simulink model "multi_model"  (R2016b)
settings: Solver=ode15s  StartTime=0.0  StopTime=inf  FixedStep=0.001  MaxStep=0.004  RelTol=1e-3
InitFcn:
  | kR_old=0;
  | kOm_old=0;
undefined symbols (not defined in the file): deg, rad, s
libraries: simulink x23, aerolibconvert2 x3, aerolibobsolete x1, aerolibtransform2 x1, aerolibatmos2 x1, aerolibnav x1, aerolibanimutils x1
(part 1 of 2)
settings Model: Creator=ADAM  LastModifiedBy=luminghua
settings SolverCC: ExtrapolationOrder=1
settings DataIOCC: MaxDataPoints=1  SaveFormat=Structure  SignalLoggingSaveFormat=ModelDataLogs  SaveOutput=off  SignalLogging=off  DSMLogging=off  SaveTime=off  OutputSaveName=model_out  SignalLoggingName=model_out
settings OptimizationCC: ExpressionDepthLimit=2147483647  LifeSpan=inf  SimCompilerOptimization=on
settings DebuggingCC: UnderspecifiedInitializationDetection=Classic  MergeDetectMultiDrivingBlocksExec=none  SolverPrmCheckMsg=warning  InheritedTsInSrcMsg=none  MultiTaskDSMMsg=warning  MultiTaskCondExecSysMsg=none  FcnCallInpInsideContextMsg=warning  UnconnectedInputMsg=none  UnconnectedOutputMsg=none  UnconnectedLineMsg=none  AllowSymbolicDim=off  StateNameClashWarn=warning  SFUnexpectedBacktrackingDiag=warning  SFNoUnconditionalDefaultTransitionDiag=warning  SFExecutionAtInitializationDiag=none
settings HardwareCC: ProdBitPerPointer=32  ProdBitPerSizeT=32  ProdBitPerPtrDiffT=32  ProdLargestAtomicFloat=None  ProdWordSize=32  ProdHWDeviceType=Generic->32-bit x86 compatible
settings ModelReferenceCC: PropagateSignalLabelsOutOfModel=off
settings CodeAppCC: MaxIdLength=95
settings GRTTargetCC: TargetLangStandard=C89/C90 (ANSI)  GeneratePreprocessorConditionals=Disable all
settings ConfigComp: CovMetricSettings=dw  CovHtmlReporting=on  CovSaveCumulativeToWorkspaceVar=on  CovSaveSingleToWorkspaceVar=on  CovExternalEMLEnable=off

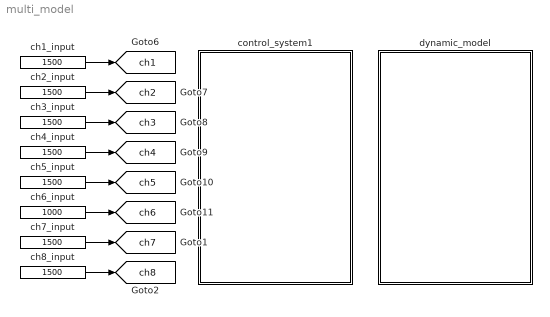
== system multi_model ==
  ch1_input : Constant  Value=1500  SampleTime=0.004
  ch2_input : Constant  Value=1500  SampleTime=0.004
  ch3_input : Constant  Value=1500  SampleTime=0.004
  ch4_input : Constant  Value=1500  SampleTime=0.004
  ch5_input : Constant  Value=1500  SampleTime=0.004
  ch6_input : Constant  Value=1000  SampleTime=0.004
  ch7_input : Constant  Value=1500  SampleTime=0.004
  ch8_input : Constant  Value=1500  SampleTime=0.004
  control_system1 : Subsystem
      mask Display: fprintf('Embedded Software')
  dynamic_model : Subsystem
      mask Display: fprintf('Dynamic Model');
  tag scope: ch1=global, ch2=global, ch3=global, ch4=global, ch5=global, ch6=global, ch7=global, ch8=global
  wires:
  ch3_input/1 -> [ch3]
  ch2_input/1 -> [ch2]
  ch1_input/1 -> [ch1]
  ch4_input/1 -> [ch4]
  ch5_input/1 -> [ch5]
  ch6_input/1 -> [ch6]
  ch7_input/1 -> [ch7]
  ch8_input/1 -> [ch8]

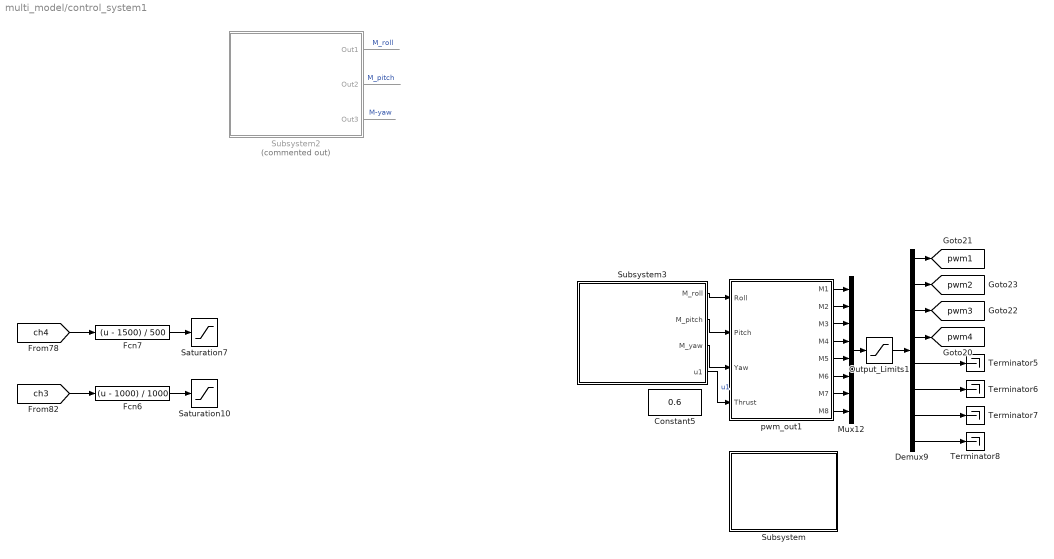
== system multi_model/control_system1 ==
  Constant5 : Constant  Value=0.6  SampleTime=0.004
  Demux9 : Demux  Outputs=8
  Fcn6 : Fcn  Expr=(u - 1000) / 1000
  Fcn7 : Fcn  Expr=(u - 1500) / 500
  Mux12 : Mux  Inputs=8
  Output_Limits1 : Saturate  UpperLimit=2000  LowerLimit=1000
  Saturation10 : Saturate  UpperLimit=1  LowerLimit=0
  Saturation7 : Saturate  UpperLimit=1  LowerLimit=-1
  Subsystem : Subsystem
      mask Display: disp('Test')
  Subsystem2 : Subsystem  Commented=on
      mask Display: disp( 'Attitude_controller  PID')
  Subsystem3 : Subsystem
      mask Display: disp('Attitude_controller distur');
  Terminator{5..8} (4 alike) : Terminator
  pwm_out1 : MATLAB Function  TreatAsAtomicUnit=on  SystemSampleTime=0.004
  tag scope: pwm1=global, pwm2=global, pwm3=global, pwm4=global
  wires:
  pwm_out1/8(M8) -> Mux12/8
  pwm_out1/7(M7) -> Mux12/7
  pwm_out1/6(M6) -> Mux12/6
  pwm_out1/5(M5) -> Mux12/5
  pwm_out1/4(M4) -> Mux12/4
  pwm_out1/3(M3) -> Mux12/3
  pwm_out1/2(M2) -> Mux12/2
  pwm_out1/1(M1) -> Mux12/1
  Mux12/1 -> Output_Limits1/1
  [ch4] -> Fcn7/1
  Fcn7/1 -> Saturation7/1
  Demux9/5 -> Terminator5/1
  Demux9/6 -> Terminator6/1
  Demux9/7 -> Terminator7/1
  Demux9/8 -> Terminator8/1
  Demux9/1 -> [pwm1]
  Demux9/2 -> [pwm2]
  Demux9/3 -> [pwm3]
  Demux9/4 -> [pwm4]
  [ch3] -> Fcn6/1
  Fcn6/1 -> Saturation10/1
  Output_Limits1/1 -> Demux9/1
  Subsystem3/4(u1) -> pwm_out1/4(Thrust)  "u1"
  Subsystem2/1(Out1) -> ?  "M_roll"
  Subsystem2/2(Out2) -> ?  "M_pitch"
  Subsystem2/3(Out3) -> ?  "M-yaw"
  Subsystem3/1(M_roll) -> pwm_out1/1(Roll)
  Subsystem3/2(M_pitch) -> pwm_out1/2(Pitch)
  Subsystem3/3(M_yaw) -> pwm_out1/3(Yaw)

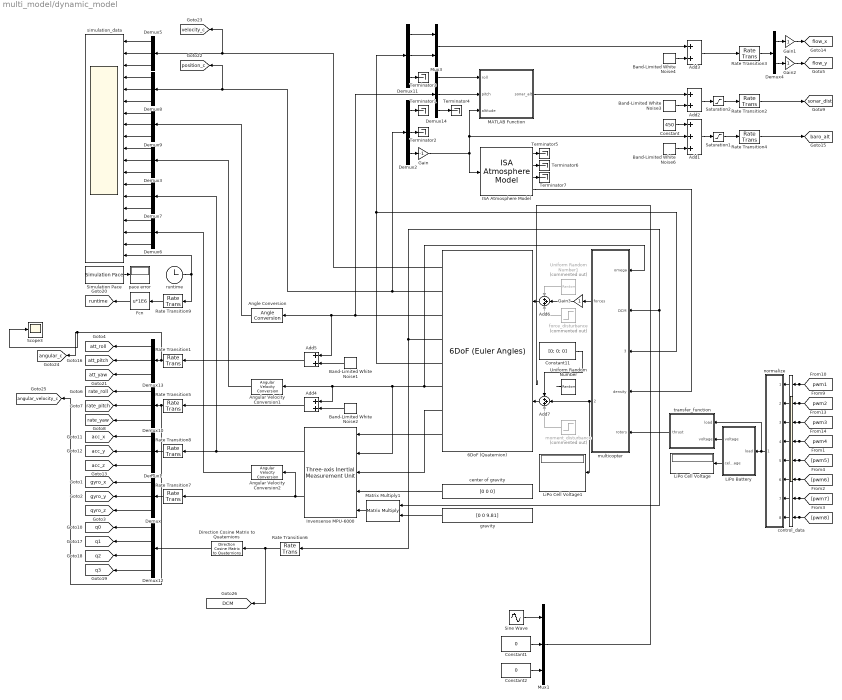
== system multi_model/dynamic_model ==
  6DoF (Quaternion) : aerolibobsolete/6DoF (Euler Angles)  units=Metric (MKS)  mtype=Fixed  rep=Quaternion  xme_0=[0 0 0]  Vm_0=[0 0 0]  eul_0=[0 0 0]  pm_0=[0 0 0]  mass_0=0.26  mass_e=0  mass_f=0  inertia=[0.00080, 0, 0; 0, 0.00065, 0; 0, 0, 0.0014]  inertia_e=eye(3)  inertia_f=eye(3)  k_quat=1.0
  Add1 : Sum  Inputs=+++
  Add{2..5} (4 alike) : Sum
  Add6 : Sum  Inputs=+++
  Add7 : Sum  Inputs=+++
  Angle Conversion : aerolibconvert2/Angle Conversion  IU=rad  OU=deg
  Angular Velocity Conversion1 : aerolibconvert2/Angular Velocity Conversion  IU=rad/s  OU=deg/s
  Angular Velocity Conversion2 : aerolibconvert2/Angular Velocity Conversion  IU=rad/s  OU=deg/s
  Band-Limited White Noise1 : simulink/Sources/Band-Limited White Noise  Cov=0.00000000015  Ts=0.004  seed=[243584]
  Band-Limited White Noise2 : simulink/Sources/Band-Limited White Noise  Cov=0.000000002  Ts=0.004  seed=[243584]
  Band-Limited White Noise3 : simulink/Sources/Band-Limited White Noise  Cov=0.000005  Ts=0.1  seed=[31841]
  Band-Limited White Noise4 : simulink/Sources/Band-Limited White Noise  Cov=0.000000003  Ts=0.0067  seed=[25481]
  Band-Limited White Noise6 : simulink/Sources/Band-Limited White Noise  Cov=0.0005  Ts=0.008  seed=[79648]
  Constant : Constant  Value=450
  Constant1 : Constant  Value=0  SampleTime=0.004
  Constant11 : Constant  Value=[0; 0; 0]  SampleTime=5
  Constant2 : Constant  Value=0  SampleTime=0.004
  Demux{,1..3,5..11,13..14} (13 alike) : Demux  Outputs=3
  Demux12 : Demux
  Demux4 : Demux  Outputs=2
  Direction Cosine Matrix to Quaternions : aerolibtransform2/Direction Cosine Matrix  to Quaternions
  Fcn : Fcn  Expr=u*1E6
      mask Display: fprintf('uS');
  Gain : Gain  Gain=-1
  Gain1 : Gain
  Gain2 : Gain
  Gain3 : Gain
  ISA Atmosphere Model : aerolibatmos2/ISA Atmosphere Model  custom=on  g=9.80665  gamma=1.4  R=287.0531  L=0.0065  h_trop=11000  h_strat=20000  rho0=1.225  P0=101325  T0=288.15  h0=0
  Invensense MPU-6000 : aerolibnav/Three-axis Inertial Measurement Unit  units=Metric (MKS)  imu=[0 0 0]  i_Ts=0.004  dtype_a=off  w_a=190  z_a=0.707  a_sf_cc=[0.98 0 0; 0 0.98 0; 0 0 0.98]  a_bias=[0 0 0]  a_sat="[-19.62  -19.62  -19.62 19.62 19.62 19.62]"  dtype_g=off  w_g=190  z_g=0.707  g_sf_cc=[.98 0 0; 0 .98 0; 0 0 .98]  g_bias=[0 0 0]  g_sens=[0 0 0]  g_sat="[-4.36  -4.36  -4.36 4.36 4.36 4.36]"  i_rand=on  i_seeds=[348631 366719 978432 189621 128794 214632]  i_pow=[0.0000005 0.0000005 0.0000005 0.000000002 0.000000002 0.000000002]
  LiPo Battery : MATLAB Function  TreatAsAtomicUnit=on  SystemSampleTime=0.004
  LiPo Cell Voltage : Display
  LiPo Cell Voltage1 : Display
  MATLAB Function : MATLAB Function  TreatAsAtomicUnit=on
  Matrix Multiply1 : Product  Multiplication=Matrix(*)
  Mux1 : Mux  Inputs=3
  Mux3 : Mux  Inputs=2
  Rate Transition{1,5..9} (6 alike) : RateTransition  OutPortSampleTime=0.004
  Rate Transition2 : RateTransition  OutPortSampleTime=0.1
  Rate Transition3 : RateTransition  OutPortSampleTime=0.0067
  Rate Transition4 : RateTransition  OutPortSampleTime=0.008
  Saturation1 : Saturate  UpperLimit=inf  LowerLimit=0
  Saturation2 : Saturate  UpperLimit=5  LowerLimit=0.3
  Scope3 : Scope
  Simulation Pace : aerolibanimutils/Simulation Pace  SimulationPace=1  SleepMode=MATLAB Thread  OutputPaceError=on  SampleTime=0.004
      settings: AttributesFormatString=%<SimulationPace> sec/sec
  Sine Wave : Sin  Amplitude=0.5  Frequency=0.01  SampleTime=0.004
  Terminator{1..7} (7 alike) : Terminator
  Uniform Random Number : UniformRandomNumber  Minimum=[-0.0005 -0.0005 -0.0001]  Maximum=[0.5 0.0005 0.0001]  SampleTime=5
  Uniform Random Number1 : UniformRandomNumber  Commented=on  Minimum=[-0.01 -0.01 -0.1]  Maximum=[0.01 0.01 0.1]  SampleTime=5
  center of gravity : Constant  Value=[0 0 0]
  control_data : Scope  NumInputPorts=8
  force_disturbance : Step  Commented=on  Time=5  Before=[0 0 0]  After=[0 0 0]
  gravity : Constant  Value=[0 0 9.81]
  moment_disturbance : Step  Commented=on  Time=5  Before=[0 0 0]  After=[0 0 0]
  multicopter : MATLAB Function  TreatAsAtomicUnit=on
  normalize : Subsystem
      mask Display:
      | port_label('input', 1, 'pwm1');
      | port_label('input', 2, 'pwm2');
      | port_label('input', 3, 'pwm3');
      | port_label('input', 4, 'pwm4');
      | port_label('input', 5, 'pwm5');
      | port_label('input', 6, 'pwm6');
      | port_label('input', 7, 'pwm7');
      | port_label('input', 8, 'pwm8');
  pace error : Display
  runtime : Clock
  simulation_data : Scope  NumInputPorts=19
  transfer_function : Subsystem
      mask Display: fprintf('Brushless Motors')
  tag scope: DCM=global, acc_x=global, acc_y=global, acc_z=global, angular_c=global, angular_velocity_c=global, att_pitch=global, att_roll=global, att_yaw=global, baro_alt=global, flow_x=global, flow_y=global, gyro_x=global, gyro_y=global, position_c=global, q0=global, q1=global, q2=global, q3=global, qyro_z=global, rate_pitch=global, rate_roll=global, rate_yaw=global, runtime=global, sonar_dist=global, velocity_c=global
  wires:
  6DoF (Quaternion)/7 -> Invensense MPU-6000/3
  Demux1/1 -> [acc_x]
  6DoF (Quaternion)/3 -> Demux14/1, Angle Conversion/1, Add5/1
  6DoF (Quaternion)/8 -> Invensense MPU-6000/1
  6DoF (Quaternion)/5 -> Demux11/1, multicopter/3(velocity)
  Demux9/1 -> simulation_data/7
  Demux9/2 -> simulation_data/8
  Demux3/1 -> simulation_data/10
  Demux3/2 -> simulation_data/11
  Demux3/3 -> simulation_data/12
  Demux7/1 -> simulation_data/13
  Demux7/2 -> simulation_data/14
  Demux7/3 -> simulation_data/15
  Demux/1 -> [gyro_x]
  Demux/2 -> [gyro_y]
  Demux/3 -> [qyro_z]
  Demux1/2 -> [acc_y]
  Demux5/1 -> simulation_data/1
  Demux5/2 -> simulation_data/2
  Demux5/3 -> simulation_data/3
  Demux8/1 -> simulation_data/4
  Demux8/2 -> simulation_data/5
  Demux8/3 -> simulation_data/6
  6DoF (Quaternion)/6 -> multicopter/1(omega), Invensense MPU-6000/2, Add4/1, Angular Velocity Conversion1/1
  Demux9/3 -> simulation_data/9
  Demux6/1 -> simulation_data/16
  Demux6/2 -> simulation_data/17
  Demux6/3 -> simulation_data/18
  Angular Velocity Conversion2/1 -> Demux6/1
  Demux1/3 -> [acc_z]
  Demux10/1 -> [rate_roll]
  Demux10/2 -> [rate_pitch]
  Demux10/3 -> [rate_yaw]
  Band-Limited White Noise2/1 -> Add4/2
  Add4/1 -> Rate Transition5/1
  Rate Transition5/1 -> [angular_velocity_c], Demux10/1
  6DoF (Quaternion)/4 -> Rate Transition6/1, Matrix Multiply1/1, multicopter/2(DCM)
  Simulation Pace/1 -> pace error/1
  6DoF (Quaternion)/1 -> Demux5/1, [velocity_c]
  6DoF (Quaternion)/2 -> Demux2/1, Demux8/1, [position_c]
  Angle Conversion/1 -> Demux9/1
  Angular Velocity Conversion1/1 -> Demux3/1
  Invensense MPU-6000/1 -> Rate Transition8/1, Demux7/1
  Invensense MPU-6000/2 -> Rate Transition7/1, Angular Velocity Conversion2/1
  runtime/1 -> simulation_data/19, Rate Transition9/1
  Rate Transition7/1 -> Demux/1
  Rate Transition8/1 -> Demux1/1
  Direction Cosine Matrix to Quaternions/1 -> Demux12/1
  [pwm1] -> normalize/1(pwm1), control_data/1
  [pwm2] -> normalize/2(pwm2), control_data/2
  [pwm3] -> normalize/3(pwm3), control_data/3
  [pwm4] -> normalize/4(pwm4), control_data/4
  [pwm5] -> normalize/5(pwm5), control_data/5
  [pwm6] -> normalize/6(pwm6), control_data/6
  [pwm7] -> normalize/7(pwm7), control_data/7
  [pwm8] -> normalize/8(pwm8), control_data/8
  Demux12/4 -> [q3]
  Demux12/3 -> [q2]
  Demux12/2 -> [q1]
  Demux12/1 -> [q0]
  Fcn/1 -> [runtime]
  Rate Transition9/1 -> Fcn/1
  normalize/1(normalized_signals) -> transfer_function/1(load), LiPo Battery/1(load)
  LiPo Battery/1(voltage) -> transfer_function/2(voltage)
  transfer_function/1(thrust) -> multicopter/5(rotors)
  LiPo Battery/2(cell_voltage) -> LiPo Cell Voltage/1
  Demux13/1 -> [att_roll]
  Demux13/2 -> [att_pitch]
  Demux13/3 -> [att_yaw]
  Rate Transition1/1 -> Scope3/1, [angular_c], Demux13/1
  Band-Limited White Noise1/1 -> Add5/2
  Add5/1 -> Rate Transition1/1
  Add6/1 -> 6DoF (Quaternion)/1
  Add7/1 -> 6DoF (Quaternion)/2
  center of gravity/1 -> Invensense MPU-6000/4
  gravity/1 -> Matrix Multiply1/2
  Matrix Multiply1/1 -> Invensense MPU-6000/5
  moment_disturbance/1 -> Add7/3
  force_disturbance/1 -> Add6/3
  multicopter/1(forces) -> Gain3/1
  Uniform Random Number1/1 -> Add6/1
  Uniform Random Number/1 -> ?
  Rate Transition3/1 -> Demux4/1
  Add3/1 -> Rate Transition3/1
  Demux2/3 -> Gain/1
  Gain/1 -> ISA Atmosphere Model/1, MATLAB Function/3(altitude), Add1/2
  Demux2/2 -> Terminator2/1
  Demux2/1 -> Terminator1/1
  Demux11/1 -> Mux3/1
  Demux11/2 -> Mux3/2
  Demux11/3 -> Terminator3/1
  Rate Transition2/1 -> [sonar_dist]
  Rate Transition4/1 -> [baro_alt]
  Saturation1/1 -> Rate Transition4/1
  Saturation2/1 -> Rate Transition2/1
  Add1/1 -> Saturation1/1
  MATLAB Function/1(sonar_alt) -> Add2/1
  Band-Limited White Noise3/1 -> Add2/2
  Add2/1 -> Saturation2/1
  Band-Limited White Noise4/1 -> Add3/2
  Band-Limited White Noise6/1 -> Add1/3
  Constant/1 -> Add1/1
  Mux3/1 -> Add3/1
  Demux4/2 -> Gain2/1
  Demux4/1 -> Gain1/1
  Gain1/1 -> [flow_x]
  Gain2/1 -> [flow_y]
  Demux14/2 -> MATLAB Function/2(pitch)
  Demux14/1 -> MATLAB Function/1(roll)
  Demux14/3 -> Terminator4/1
  ISA Atmosphere Model/3 -> Terminator7/1
  ISA Atmosphere Model/2 -> Terminator6/1
  ISA Atmosphere Model/1 -> Terminator5/1
  ISA Atmosphere Model/4 -> multicopter/4(density)
  Constant11/1 -> Add7/1
  multicopter/2(moments) -> Add7/2, LiPo Cell Voltage1/1
  Gain3/1 -> Add6/2
  Sine Wave/1 -> Mux1/1
  Constant1/1 -> Mux1/2
  Constant2/1 -> Mux1/3
  Mux1/1 -> ?
  Rate Transition6/1 -> [DCM], Direction Cosine Matrix to Quaternions/1

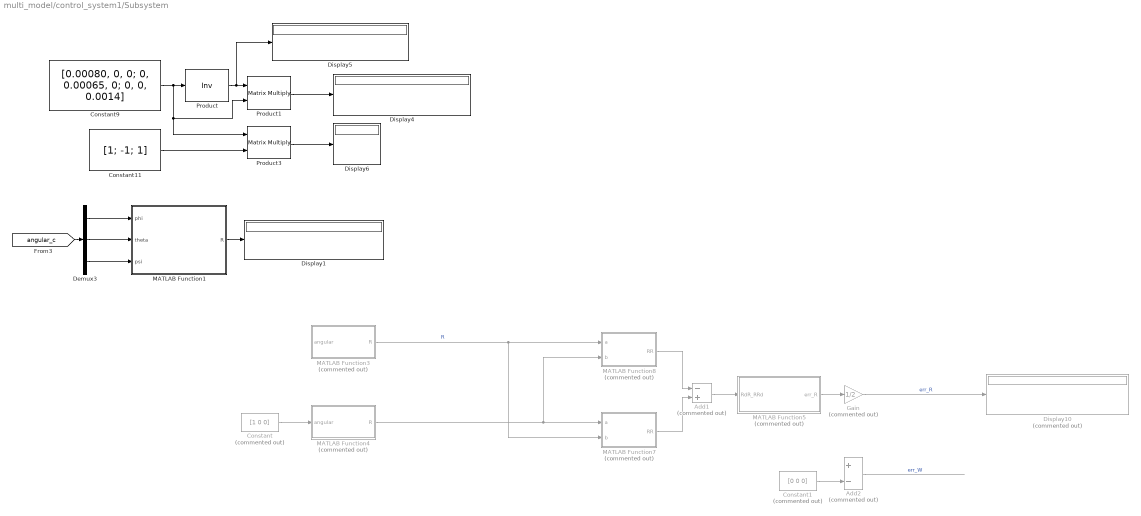
== system multi_model/control_system1/Subsystem ==
  Add1 : Sum  Commented=on  Inputs=-+
  Add2 : Sum  Commented=on  Inputs=+-
  Constant : Constant  Commented=on  Value=[1 0 0]
  Constant1 : Constant  Commented=on  Value=[0 0 0]
  Constant11 : Constant  Value=[1; -1; 1]  SampleTime=0.004
  Constant9 : Constant  Value=[0.00080, 0, 0; 0, 0.00065, 0; 0, 0, 0.0014]  SampleTime=0.004
  Demux3 : Demux  Outputs=3
  Display{1,4..6} (4 alike) : Display
  Display10 : Display  Commented=on
  Gain : Gain  Commented=on  Gain=1/2
  MATLAB Function1 : MATLAB Function  TreatAsAtomicUnit=on
  MATLAB Function3 : MATLAB Function  Commented=on  TreatAsAtomicUnit=on
  MATLAB Function4 : MATLAB Function  Commented=on  TreatAsAtomicUnit=on
  MATLAB Function5 : MATLAB Function  Commented=on  TreatAsAtomicUnit=on
  MATLAB Function7 : MATLAB Function  Commented=on  TreatAsAtomicUnit=on
  MATLAB Function8 : MATLAB Function  Commented=on  TreatAsAtomicUnit=on
  Product : Product  Inputs=/  Multiplication=Matrix(*)
  Product1 : Product  Multiplication=Matrix(*)
  Product3 : Product  Multiplication=Matrix(*)
  wires:
  ? -> Add2/1
  ? -> MATLAB Function3/1(angular)
  MATLAB Function7/1(RR) -> Add1/2
  Add1/1 -> MATLAB Function5/1(RdR_RRd)
  Constant/1 -> MATLAB Function4/1(angular)
  Gain/1 -> Display10/1  "err_R"
  MATLAB Function3/1(R) -> MATLAB Function8/1(a), MATLAB Function7/2(b)  "R"
  MATLAB Function5/1(err_R) -> Gain/1
  MATLAB Function8/1(RR) -> Add1/1
  MATLAB Function4/1(R) -> MATLAB Function8/2(b), MATLAB Function7/1(a)
  Constant1/1 -> Add2/2
  Product/1 -> Product1/1, Display5/1
  Constant11/1 -> Product3/2
  Constant9/1 -> Product3/1, Product1/2, Product/1
  Add2/1 -> ?  "err_W"
  Product3/1 -> Display6/1
  Product1/1 -> Display4/1
  MATLAB Function1/1(R) -> Display1/1
  Demux3/2 -> MATLAB Function1/2(theta)
  Demux3/1 -> MATLAB Function1/1(phi)
  Demux3/3 -> MATLAB Function1/3(psi)
  [angular_c] -> Demux3/1

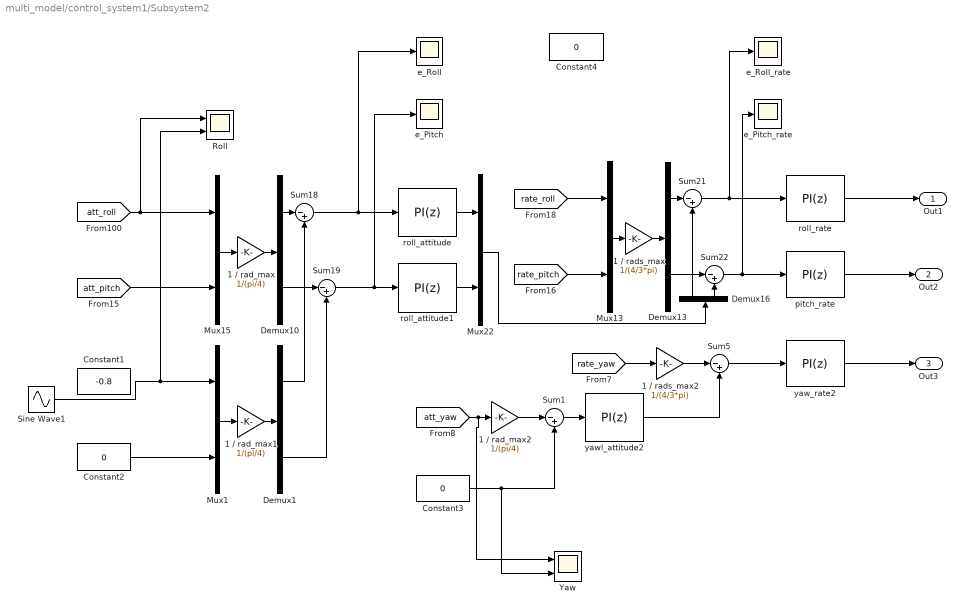
== system multi_model/control_system1/Subsystem2 ==
  1 / rad_max : Gain  Gain=1/(pi/4)
  1 / rad_max1 : Gain  Gain=1/(pi/4)
  1 / rad_max2 : Gain  Gain=1/(pi/4)
  1 / rads_max : Gain  Gain=1/(4/3*pi)
  1 / rads_max2 : Gain  Gain=1/(4/3*pi)
  Constant1 : Constant  Value=-0.8  SampleTime=0.004
  Constant2 : Constant  Value=0  SampleTime=0.004
  Constant3 : Constant  Value=0  SampleTime=0.004
  Constant4 : Constant  Value=0  SampleTime=0.004
  Demux{1,10,13,16} (4 alike) : Demux  Outputs=2
  Mux{1,13,15,22} (4 alike) : Mux  Inputs=2
  Roll : Scope  NumInputPorts=2
  Sine Wave1 : Sin  Amplitude=pi/9  Frequency=pi  Phase=pi/2  SampleTime=0.004
  Sum{1,5,18..19,21..22} (6 alike) : Sum  Inputs=|-+
  Yaw : Scope  NumInputPorts=2
  e_Pitch : Scope
  e_Pitch_rate : Scope
  e_Roll : Scope
  e_Roll_rate : Scope
  pitch_rate : simulink/Continuous/PID Controller  Controller=PI  TimeDomain=Discrete-time  SampleTime=-1  IntegratorMethod=Forward Euler  FilterMethod=Forward Euler  Form=Parallel  UseFilter=on  ControllerParametersSource=internal  P=0.266243984189179  I=1.55321106287276  D=0.0024  N=100  InitialConditionSource=internal  InitialConditionForIntegrator=0  InitialConditionForFilter=0  ExternalReset=none  LimitOutput=on  UpperSaturationLimit=1  LowerSaturationLimit=-1  LinearizeAsGain=on  AntiWindupMode=none  Kb=1  TrackingMode=off  Kt=1  PParamMin=[]  PParamMax=[]  IParamMin=[]  IParamMax=[]  DParamMin=[]  DParamMax=[]  NParamMin=[]  NParamMax=[]  KbParamMin=[]  KbParamMax=[]  KtParamMin=[]  KtParamMax=[]  POutMin=[]  POutMax=[]  IOutMin=[]  IOutMax=[]  DOutMin=[]  DOutMax=[]  NOutMin=[]  NOutMax=[]  KbOutMin=[]  KbOutMax=[]  KtOutMin=[]  KtOutMax=[]  IntegratorOutMin=[]  IntegratorOutMax=[]  FilterOutMin=[]  FilterOutMax=[]  SumOutMin=[]  SumOutMax=[]  SumI1OutMin=[]  SumI1OutMax=[]  SumI2OutMin=[]  SumI2OutMax=[]  SumI3OutMin=[]  SumI3OutMax=[]  SumDOutMin=[]  SumDOutMax=[]  SaturationOutMin=[]  SaturationOutMax=[]  IntegratorContinuousStateAttributes=''  IntegratorStateMustResolveToSignalObject=off  IntegratorRTWStateStorageClass=Auto  FilterContinuousStateAttributes=''  FilterStateMustResolveToSignalObject=off  FilterRTWStateStorageClass=Auto  DifferentiatorICPrevScaledInput=0  DifferentiatorOutMin=[]  DifferentiatorOutMax=[]
  roll_attitude : simulink/Continuous/PID Controller  Controller=PI  TimeDomain=Discrete-time  SampleTime=-1  IntegratorMethod=Forward Euler  FilterMethod=Forward Euler  Form=Parallel  UseFilter=on  ControllerParametersSource=internal  P=1.14248027715292  I=2.67479021353904  D=0.01  N=100  InitialConditionSource=internal  InitialConditionForIntegrator=0  InitialConditionForFilter=0  ExternalReset=none  LimitOutput=on  UpperSaturationLimit=1  LowerSaturationLimit=-1  LinearizeAsGain=on  AntiWindupMode=none  Kb=1  TrackingMode=off  Kt=1  PParamMin=[]  PParamMax=[]  IParamMin=[]  IParamMax=[]  DParamMin=[]  DParamMax=[]  NParamMin=[]  NParamMax=[]  KbParamMin=[]  KbParamMax=[]  KtParamMin=[]  KtParamMax=[]  POutMin=[]  POutMax=[]  IOutMin=[]  IOutMax=[]  DOutMin=[]  DOutMax=[]  NOutMin=[]  NOutMax=[]  KbOutMin=[]  KbOutMax=[]  KtOutMin=[]  KtOutMax=[]  IntegratorOutMin=[]  IntegratorOutMax=[]  FilterOutMin=[]  FilterOutMax=[]  SumOutMin=[]  SumOutMax=[]  SumI1OutMin=[]  SumI1OutMax=[]  SumI2OutMin=[]  SumI2OutMax=[]  SumI3OutMin=[]  SumI3OutMax=[]  SumDOutMin=[]  SumDOutMax=[]  SaturationOutMin=[]  SaturationOutMax=[]  IntegratorContinuousStateAttributes=''  IntegratorStateMustResolveToSignalObject=off  IntegratorRTWStateStorageClass=Auto  FilterContinuousStateAttributes=''  FilterStateMustResolveToSignalObject=off  FilterRTWStateStorageClass=Auto  DifferentiatorICPrevScaledInput=0  DifferentiatorOutMin=[]  DifferentiatorOutMax=[]
  roll_attitude1 : simulink/Continuous/PID Controller  Controller=PI  TimeDomain=Discrete-time  SampleTime=-1  IntegratorMethod=Forward Euler  FilterMethod=Forward Euler  Form=Parallel  UseFilter=on  ControllerParametersSource=internal  P=1.14248027709528  I=2.67479021340165  D=0.01  N=100  InitialConditionSource=internal  InitialConditionForIntegrator=0  InitialConditionForFilter=0  ExternalReset=none  LimitOutput=on  UpperSaturationLimit=1  LowerSaturationLimit=-1  LinearizeAsGain=on  AntiWindupMode=none  Kb=1  TrackingMode=off  Kt=1  PParamMin=[]  PParamMax=[]  IParamMin=[]  IParamMax=[]  DParamMin=[]  DParamMax=[]  NParamMin=[]  NParamMax=[]  KbParamMin=[]  KbParamMax=[]  KtParamMin=[]  KtParamMax=[]  POutMin=[]  POutMax=[]  IOutMin=[]  IOutMax=[]  DOutMin=[]  DOutMax=[]  NOutMin=[]  NOutMax=[]  KbOutMin=[]  KbOutMax=[]  KtOutMin=[]  KtOutMax=[]  IntegratorOutMin=[]  IntegratorOutMax=[]  FilterOutMin=[]  FilterOutMax=[]  SumOutMin=[]  SumOutMax=[]  SumI1OutMin=[]  SumI1OutMax=[]  SumI2OutMin=[]  SumI2OutMax=[]  SumI3OutMin=[]  SumI3OutMax=[]  SumDOutMin=[]  SumDOutMax=[]  SaturationOutMin=[]  SaturationOutMax=[]  IntegratorContinuousStateAttributes=''  IntegratorStateMustResolveToSignalObject=off  IntegratorRTWStateStorageClass=Auto  FilterContinuousStateAttributes=''  FilterStateMustResolveToSignalObject=off  FilterRTWStateStorageClass=Auto  DifferentiatorICPrevScaledInput=0  DifferentiatorOutMin=[]  DifferentiatorOutMax=[]
  roll_rate : simulink/Continuous/PID Controller  Controller=PI  TimeDomain=Discrete-time  SampleTime=-1  IntegratorMethod=Forward Euler  FilterMethod=Forward Euler  Form=Parallel  UseFilter=on  ControllerParametersSource=internal  P=0.327684903617463  I=1.91164438507472  D=0.0024  N=100  InitialConditionSource=internal  InitialConditionForIntegrator=0  InitialConditionForFilter=0  ExternalReset=none  LimitOutput=on  UpperSaturationLimit=1  LowerSaturationLimit=-1  LinearizeAsGain=on  AntiWindupMode=none  Kb=1  TrackingMode=off  Kt=1  PParamMin=[]  PParamMax=[]  IParamMin=[]  IParamMax=[]  DParamMin=[]  DParamMax=[]  NParamMin=[]  NParamMax=[]  KbParamMin=[]  KbParamMax=[]  KtParamMin=[]  KtParamMax=[]  POutMin=[]  POutMax=[]  IOutMin=[]  IOutMax=[]  DOutMin=[]  DOutMax=[]  NOutMin=[]  NOutMax=[]  KbOutMin=[]  KbOutMax=[]  KtOutMin=[]  KtOutMax=[]  IntegratorOutMin=[]  IntegratorOutMax=[]  FilterOutMin=[]  FilterOutMax=[]  SumOutMin=[]  SumOutMax=[]  SumI1OutMin=[]  SumI1OutMax=[]  SumI2OutMin=[]  SumI2OutMax=[]  SumI3OutMin=[]  SumI3OutMax=[]  SumDOutMin=[]  SumDOutMax=[]  SaturationOutMin=[]  SaturationOutMax=[]  IntegratorContinuousStateAttributes=''  IntegratorStateMustResolveToSignalObject=off  IntegratorRTWStateStorageClass=Auto  FilterContinuousStateAttributes=''  FilterStateMustResolveToSignalObject=off  FilterRTWStateStorageClass=Auto  DifferentiatorICPrevScaledInput=0  DifferentiatorOutMin=[]  DifferentiatorOutMax=[]
  yaw_rate2 : simulink/Continuous/PID Controller  Controller=PI  TimeDomain=Discrete-time  SampleTime=-1  IntegratorMethod=Forward Euler  FilterMethod=Forward Euler  Form=Parallel  UseFilter=on  ControllerParametersSource=internal  P=0.3  I=0.03  D=0.0024  N=100  InitialConditionSource=internal  InitialConditionForIntegrator=0  InitialConditionForFilter=0  ExternalReset=none  LimitOutput=on  UpperSaturationLimit=1  LowerSaturationLimit=-1  LinearizeAsGain=on  AntiWindupMode=none  Kb=1  TrackingMode=off  Kt=1  PParamMin=[]  PParamMax=[]  IParamMin=[]  IParamMax=[]  DParamMin=[]  DParamMax=[]  NParamMin=[]  NParamMax=[]  KbParamMin=[]  KbParamMax=[]  KtParamMin=[]  KtParamMax=[]  POutMin=[]  POutMax=[]  IOutMin=[]  IOutMax=[]  DOutMin=[]  DOutMax=[]  NOutMin=[]  NOutMax=[]  KbOutMin=[]  KbOutMax=[]  KtOutMin=[]  KtOutMax=[]  IntegratorOutMin=[]  IntegratorOutMax=[]  FilterOutMin=[]  FilterOutMax=[]  SumOutMin=[]  SumOutMax=[]  SumI1OutMin=[]  SumI1OutMax=[]  SumI2OutMin=[]  SumI2OutMax=[]  SumI3OutMin=[]  SumI3OutMax=[]  SumDOutMin=[]  SumDOutMax=[]  SaturationOutMin=[]  SaturationOutMax=[]  IntegratorContinuousStateAttributes=''  IntegratorStateMustResolveToSignalObject=off  IntegratorRTWStateStorageClass=Auto  FilterContinuousStateAttributes=''  FilterStateMustResolveToSignalObject=off  FilterRTWStateStorageClass=Auto  DifferentiatorICPrevScaledInput=0  DifferentiatorOutMin=[]  DifferentiatorOutMax=[]
  yawl_attitude2 : simulink/Continuous/PID Controller  Controller=PI  TimeDomain=Discrete-time  SampleTime=-1  IntegratorMethod=Forward Euler  FilterMethod=Forward Euler  Form=Parallel  UseFilter=on  ControllerParametersSource=internal  P=0.5  I=0.05  D=0.01  N=100  InitialConditionSource=internal  InitialConditionForIntegrator=0  InitialConditionForFilter=0  ExternalReset=none  LimitOutput=on  UpperSaturationLimit=1  LowerSaturationLimit=-1  LinearizeAsGain=on  AntiWindupMode=none  Kb=1  TrackingMode=off  Kt=1  PParamMin=[]  PParamMax=[]  IParamMin=[]  IParamMax=[]  DParamMin=[]  DParamMax=[]  NParamMin=[]  NParamMax=[]  KbParamMin=[]  KbParamMax=[]  KtParamMin=[]  KtParamMax=[]  POutMin=[]  POutMax=[]  IOutMin=[]  IOutMax=[]  DOutMin=[]  DOutMax=[]  NOutMin=[]  NOutMax=[]  KbOutMin=[]  KbOutMax=[]  KtOutMin=[]  KtOutMax=[]  IntegratorOutMin=[]  IntegratorOutMax=[]  FilterOutMin=[]  FilterOutMax=[]  SumOutMin=[]  SumOutMax=[]  SumI1OutMin=[]  SumI1OutMax=[]  SumI2OutMin=[]  SumI2OutMax=[]  SumI3OutMin=[]  SumI3OutMax=[]  SumDOutMin=[]  SumDOutMax=[]  SaturationOutMin=[]  SaturationOutMax=[]  IntegratorContinuousStateAttributes=''  IntegratorStateMustResolveToSignalObject=off  IntegratorRTWStateStorageClass=Auto  FilterContinuousStateAttributes=''  FilterStateMustResolveToSignalObject=off  FilterRTWStateStorageClass=Auto  DifferentiatorICPrevScaledInput=0  DifferentiatorOutMin=[]  DifferentiatorOutMax=[]
  Out1 : Outport
  Out2 : Outport  Port=2
  Out3 : Outport  Port=3
  wires:
  Sine Wave1/1 -> Roll/2, Mux1/1
  Mux1/1 -> 1 / rad_max1/1
  Constant2/1 -> Mux1/2
  Demux1/1 -> Sum18/2
  Mux22/1 -> Demux16/1
  yaw_rate2/1 -> Out3/1
  Sum5/1 -> yaw_rate2/1
  yawl_attitude2/1 -> Sum5/2
  1 / rad_max2/1 -> Sum1/1
  [att_yaw] -> Yaw/1, 1 / rad_max2/1
  1 / rads_max2/1 -> Sum5/1
  [rate_yaw] -> 1 / rads_max2/1
  1 / rad_max/1 -> Demux10/1
  Demux10/1 -> Sum18/1
  Demux16/2 -> Sum22/2
  roll_attitude1/1 -> Mux22/2
  Demux13/2 -> Sum22/1
  Sum21/1 -> e_Roll_rate/1, roll_rate/1
  Sum22/1 -> e_Pitch_rate/1, pitch_rate/1
  roll_attitude/1 -> Mux22/1
  [rate_pitch] -> Mux13/2
  Demux10/2 -> Sum19/1
  [att_pitch] -> Mux15/2
  [rate_roll] -> Mux13/1
  1 / rads_max/1 -> Demux13/1
  Sum18/1 -> e_Roll/1, roll_attitude/1
  Mux13/1 -> 1 / rads_max/1
  Demux13/1 -> Sum21/1
  Sum19/1 -> e_Pitch/1, roll_attitude1/1
  Mux15/1 -> 1 / rad_max/1
  [att_roll] -> Roll/1, Mux15/1
  roll_rate/1 -> Out1/1
  pitch_rate/1 -> Out2/1
  1 / rad_max1/1 -> Demux1/1
  Demux1/2 -> Sum19/2
  Sum1/1 -> yawl_attitude2/1
  Constant3/1 -> Yaw/2, Sum1/2
  Demux16/1 -> Sum21/2

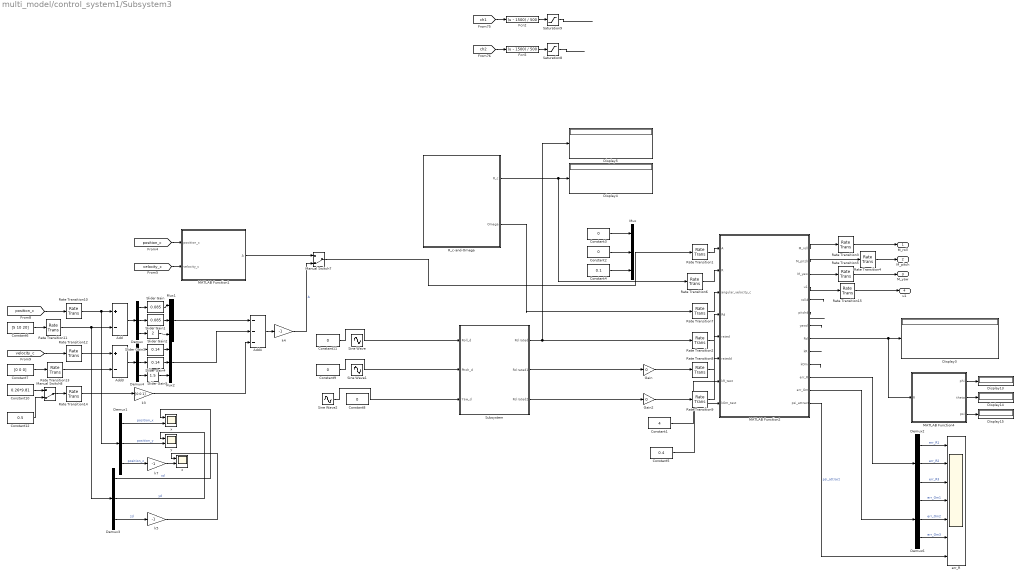
== system multi_model/control_system1/Subsystem3 ==
  Add : Sum  Inputs=+-
  Add3 : Sum  Inputs=+-
  Add4 : Sum  Inputs=---
  Constant1 : Constant  Value=4  SampleTime=0.004
  Constant10 : Constant  Value=0.26*9.81  SampleTime=0.004
  Constant{2..3,8..9,11} (5 alike) : Constant  Value=0  SampleTime=0.004
  Constant12 : Constant  Value=0.5  SampleTime=0.004
  Constant4 : Constant  Value=0.1  SampleTime=0.004
  Constant5 : Constant  Value=0.4  SampleTime=0.004
  Constant6 : Constant  Value=[5 10 20]  SampleTime=0.004
  Constant7 : Constant  Value=[0 0 0]  SampleTime=0.004
  Demux{,1..4,6} (6 alike) : Demux  Outputs=3
  Display{3..5,13..15} (6 alike) : Display
  Fcn2 : Fcn  Expr=(u - 1500) / 500
  Fcn5 : Fcn  Expr=(u - 1500) / 500
  Gain : Gain  Gain=0
  Gain2 : Gain  Gain=0
  MATLAB Function1 : MATLAB Function  TreatAsAtomicUnit=on
  MATLAB Function2 : MATLAB Function  TreatAsAtomicUnit=on
  MATLAB Function4 : MATLAB Function  TreatAsAtomicUnit=on
  Manual Switch7 : ManualSwitch  CurrentSetting=0
  Manual Switch8 : ManualSwitch  CurrentSetting=0
  Mux : Mux  Inputs=3
  Mux1 : Mux  Inputs=3
  Mux2 : Mux  Inputs=3
  R_c-and-Omega : Subsystem
  Rate Transition{1..15} (15 alike) : RateTransition  OutPortSampleTime=0.004
  Saturation8 : Saturate  UpperLimit=1  LowerLimit=-1
  Saturation9 : Saturate  UpperLimit=1  LowerLimit=-1
  Sine Wave : Sin  Amplitude=pi/9  Frequency=pi  SampleTime=0.004
  Sine Wave1 : Sin  Amplitude=pi/9  Frequency=pi  Phase=pi/2  SampleTime=0.004
  Sine Wave2 : Sin  Amplitude=pi/9  Frequency=pi  SampleTime=0.004
  Slider Gain : simulink/Math Operations/Slider Gain  low=0  gain=0.085  high=1
  Slider Gain1 : simulink/Math Operations/Slider Gain  low=0  gain=0.085  high=1
  Slider Gain2 : simulink/Math Operations/Slider Gain  low=0  gain=2  high=10
  Slider Gain3 : simulink/Math Operations/Slider Gain  low=0  gain=0.14  high=1
  Slider Gain4 : simulink/Math Operations/Slider Gain  low=0  gain=0.14  high=2
  Slider Gain5 : simulink/Math Operations/Slider Gain  low=0  gain=1.5  high=10
  Subsystem : Subsystem
  err_R : Scope  NumInputPorts=7
  k3 : Gain  Gain=[0 0 1]
  k4 : Gain  Gain=-1
  k5 : Gain  Gain=-1
  k7 : Gain  Gain=-1
  x : Scope  NumInputPorts=2
  y : Scope  NumInputPorts=2
  z : Scope  NumInputPorts=2
  M_roll : Outport
  M_pitch : Outport  Port=2
  M_yaw : Outport  Port=3
  u1 : Outport  Port=4
  wires:
  Rate Transition5/1 -> M_yaw/1
  Rate Transition4/1 -> M_pitch/1
  Rate Transition3/1 -> M_roll/1
  Rate Transition2/1 -> MATLAB Function2/4("Rd ")
  Saturation8/1 -> ?
  MATLAB Function2/3(M_yaw) -> Rate Transition5/1
  Constant11/1 -> Subsystem/1(Roll_d)
  MATLAB Function2/1(M_roll) -> Rate Transition3/1
  Saturation9/1 -> ?
  MATLAB Function2/2(M_pitch) -> Rate Transition4/1
  Subsystem/1(Rd rated) -> Rate Transition2/1, Display5/1
  Constant4/1 -> Mux/3
  Rate Transition6/1 -> MATLAB Function2/2(R)
  Rate Transition7/1 -> MATLAB Function2/3(angular_velocity_c)
  Rate Transition1/1 -> MATLAB Function2/1(A)
  R_c-and-Omega/2(Omega) -> Rate Transition7/1
  MATLAB Function2/5(rolld) -> ?
  MATLAB Function2/7(yawd) -> ?
  MATLAB Function2/6(pitchd) -> ?
  MATLAB Function2/4(u1) -> Rate Transition15/1
  Demux2/1 -> err_R/1  "err_R1"
  MATLAB Function2/9(kR) -> ?
  MATLAB Function2/10(kOm) -> ?
  Demux2/2 -> err_R/2  "err_R2"
  Demux2/3 -> err_R/3  "err_R3"
  Sine Wave2/1 -> Subsystem/3(Yaw_d)
  Constant9/1 -> Subsystem/2(PItch_d)
  MATLAB Function4/1(phi) -> Display13/1
  MATLAB Function4/2(theta) -> Display14/1
  MATLAB Function4/3(psi) -> Display15/1
  MATLAB Function2/8(Rd) -> MATLAB Function4/1(R), Display3/1
  Rate Transition8/1 -> MATLAB Function2/5(rated)
  Rate Transition9/1 -> MATLAB Function2/6(ratedd)
  Subsystem/2(Rd rated1) -> Gain/1
  Subsystem/3(Rd rated2) -> Gain2/1
  MATLAB Function2/13(psi_attract) -> err_R/7  "psi_attract"
  MATLAB Function2/11(err_R) -> Demux2/1
  Demux6/1 -> err_R/4  "err_Om1"
  Demux6/2 -> err_R/5  "err_Om2"
  Demux6/3 -> err_R/6  "err_Om3"
  MATLAB Function2/12(err_Om) -> Demux6/1
  Gain/1 -> Rate Transition8/1
  Gain2/1 -> Rate Transition9/1
  R_c-and-Omega/1(R_c) -> Rate Transition6/1, Display4/1
  Constant1/1 -> MATLAB Function2/7(kR_test)
  Constant5/1 -> MATLAB Function2/8(kOm_test)
  [ch1] -> Fcn2/1
  [ch2] -> Fcn5/1
  Fcn5/1 -> Saturation8/1
  Fcn2/1 -> Saturation9/1
  [position_c] -> MATLAB Function1/1(position_c)
  [velocity_c] -> MATLAB Function1/2(velocity_c)
  Constant6/1 -> Rate Transition11/1
  [position_c] -> Rate Transition10/1
  Constant7/1 -> Rate Transition13/1
  [velocity_c] -> Rate Transition12/1
  Add3/1 -> Demux4/1
  k3/1 -> Add4/3
  Add4/1 -> k4/1
  k4/1 -> Manual Switch7/2  "A"
  MATLAB Function1/1(A) -> Manual Switch7/1
  Demux1/1 -> x/2  "position_x"
  Demux1/2 -> y/2  "position_y"
  Demux1/3 -> k7/1  "position_z"
  Demux3/1 -> x/1  "xd"
  Demux3/2 -> y/1  "yd"
  Demux3/3 -> k5/1  "zd"
  k5/1 -> z/1
  k7/1 -> z/2
  Constant10/1 -> Manual Switch8/1
  Manual Switch8/1 -> Rate Transition14/1
  Constant12/1 -> Manual Switch8/2
  Rate Transition10/1 -> Demux1/1, Add/1
  Rate Transition11/1 -> Demux3/1, Add/2
  Rate Transition12/1 -> Add3/1
  Rate Transition13/1 -> Add3/2
  Rate Transition14/1 -> k3/1
  Demux/1 -> Slider Gain/1
  Demux/2 -> Slider Gain1/1
  Demux/3 -> Slider Gain2/1
  Add/1 -> Demux/1
  Slider Gain/1 -> Mux1/1
  Slider Gain1/1 -> Mux1/2
  Slider Gain2/1 -> Mux1/3
  Mux1/1 -> Add4/1
  Demux4/1 -> Slider Gain3/1
  Demux4/2 -> Slider Gain4/1
  Demux4/3 -> Slider Gain5/1
  Slider Gain3/1 -> Mux2/1
  Slider Gain4/1 -> Mux2/2
  Slider Gain5/1 -> Mux2/3
  Mux2/1 -> Add4/2
  Manual Switch7/1 -> Rate Transition1/1
  Constant3/1 -> Mux/1
  Constant2/1 -> Mux/2
  Rate Transition15/1 -> u1/1

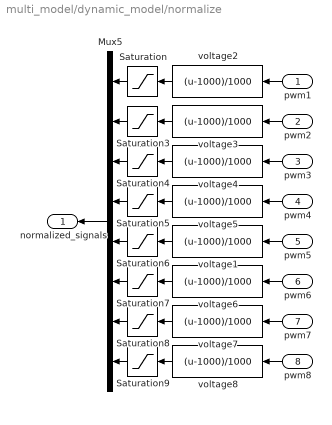
== system multi_model/dynamic_model/normalize ==
  pwm1 : Inport
  pwm2 : Inport  Port=2
  pwm3 : Inport  Port=3
  pwm4 : Inport  Port=4
  pwm5 : Inport  Port=5
  pwm6 : Inport  Port=6
  pwm7 : Inport  Port=7
  pwm8 : Inport  Port=8
  Mux5 : Mux  Inputs=8
  Saturation{,3..9} (8 alike) : Saturate  UpperLimit=1  LowerLimit=0
  voltage{1..8} (8 alike) : Fcn  Expr=(u-1000)/1000
  normalized_signals : Outport
  wires:
  Saturation5/1 -> Mux5/4
  Saturation7/1 -> Mux5/6
  voltage6/1 -> Saturation7/1
  voltage5/1 -> Saturation5/1
  voltage2/1 -> Saturation/1
  voltage7/1 -> Saturation8/1
  Saturation8/1 -> Mux5/7
  voltage8/1 -> Saturation9/1
  Saturation9/1 -> Mux5/8
  pwm3/1 -> voltage4/1
  Mux5/1 -> normalized_signals/1
  pwm1/1 -> voltage2/1
  voltage4/1 -> Saturation4/1
  Saturation4/1 -> Mux5/3
  pwm7/1 -> voltage7/1
  pwm6/1 -> voltage6/1
  pwm8/1 -> voltage8/1
  pwm4/1 -> voltage5/1
  pwm5/1 -> voltage1/1
  pwm2/1 -> voltage3/1
  voltage1/1 -> Saturation6/1
  Saturation6/1 -> Mux5/5
  Saturation/1 -> Mux5/1
  Saturation3/1 -> Mux5/2
  voltage3/1 -> Saturation3/1

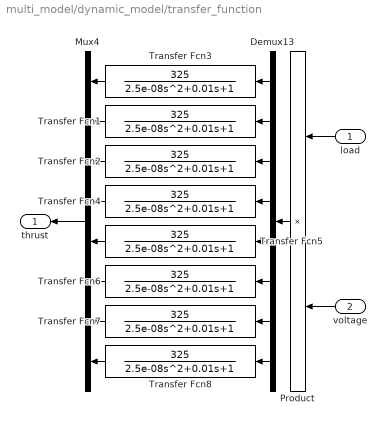
== system multi_model/dynamic_model/transfer_function ==
  load : Inport  PortDimensions=[8]
  voltage : Inport  Port=2  PortDimensions=[8]
  Demux13 : Demux  Outputs=8
  Mux4 : Mux  Inputs=8
  Product : Product
  Transfer Fcn{1..8} (8 alike) : TransferFcn  Numerator=[325]  Denominator=[2.5e-08 0.01 1]  ContinuousStateAttributes='angular_velocity'
  thrust : Outport
  wires:
  Demux13/6 -> Transfer Fcn6/1
  Transfer Fcn4/1 -> Mux4/4
  Transfer Fcn2/1 -> Mux4/3
  Demux13/8 -> Transfer Fcn8/1
  Transfer Fcn8/1 -> Mux4/8
  Transfer Fcn1/1 -> Mux4/2
  Demux13/7 -> Transfer Fcn7/1
  Transfer Fcn7/1 -> Mux4/7
  Transfer Fcn5/1 -> Mux4/5
  Demux13/5 -> Transfer Fcn5/1
  Transfer Fcn3/1 -> Mux4/1
  Transfer Fcn6/1 -> Mux4/6
  Demux13/1 -> Transfer Fcn3/1
  Demux13/2 -> Transfer Fcn1/1
  Demux13/3 -> Transfer Fcn2/1
  Demux13/4 -> Transfer Fcn4/1
  voltage/1 -> Product/2
  Product/1 -> Demux13/1
  Mux4/1 -> thrust/1
  load/1 -> Product/1

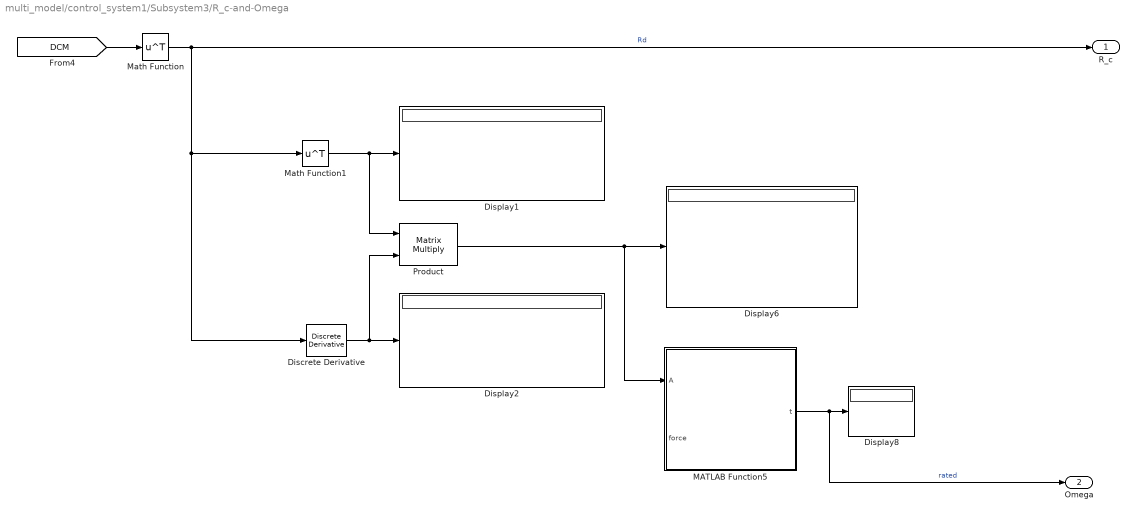
== system multi_model/control_system1/Subsystem3/R_c-and-Omega ==
  Discrete Derivative : simulink/Discrete/Discrete Derivative  gainval=1.0  ICPrevScaledInput=0.0  OutMin=[]  OutMax=[]  OutDataType=fixdt(1, 16)  OutScaling=2^-10  DoSatur=off
  Display{1..2,6,8} (4 alike) : Display
  MATLAB Function5 : MATLAB Function  TreatAsAtomicUnit=on
  Math Function : Math  Operator=transpose  SaturateOnIntegerOverflow=on
  Math Function1 : Math  Operator=transpose  SaturateOnIntegerOverflow=on
  Product : Product  Multiplication=Matrix(*)
  R_c : Outport
  Omega : Outport  Port=2
  wires:
  [DCM] -> Math Function/1
  Product/1 -> MATLAB Function5/1(A), Display6/1
  Math Function1/1 -> Product/1, Display1/1
  Discrete Derivative/1 -> Product/2, Display2/1
  MATLAB Function5/1(t) -> Omega/1, Display8/1  "rated"
  ? -> MATLAB Function5/2(force)
  Math Function/1 -> R_c/1, Math Function1/1, Discrete Derivative/1  "Rd"

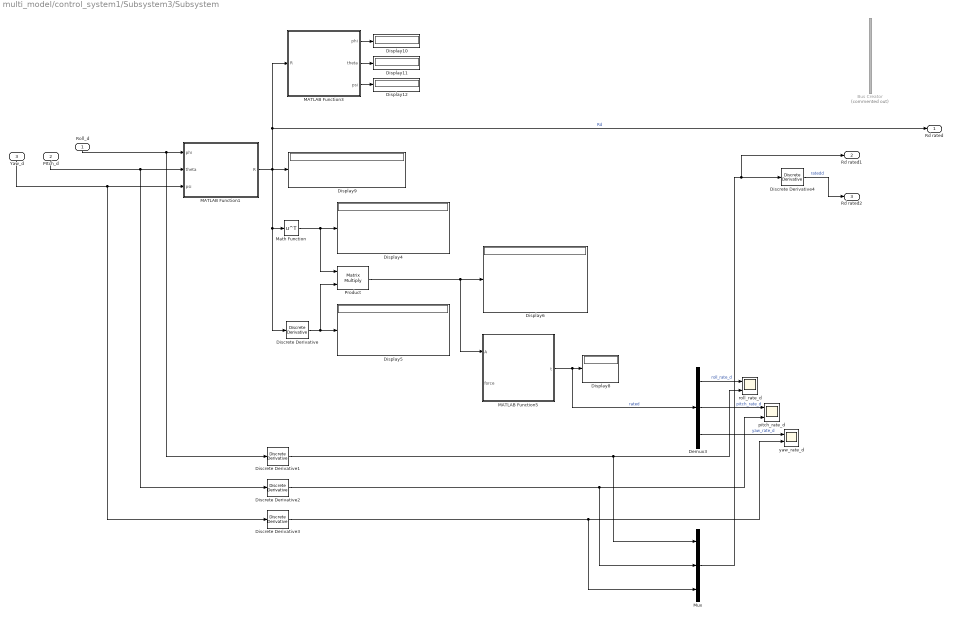
== system multi_model/control_system1/Subsystem3/Subsystem ==
  Roll_d : Inport
  PItch_d : Inport  Port=2
  Yaw_d : Inport  Port=3
  Bus Creator : BusCreator  Commented=on  Inputs=3
  Demux3 : Demux  Outputs=3
  Discrete Derivative{,1..4} (5 alike) : simulink/Discrete/Discrete Derivative  gainval=1.0  ICPrevScaledInput=0.0  OutMin=[]  OutMax=[]  OutDataType=fixdt(1, 16)  OutScaling=2^-10  DoSatur=off
  Display{4..6,8..12} (8 alike) : Display
  MATLAB Function1 : MATLAB Function  TreatAsAtomicUnit=on
  MATLAB Function3 : MATLAB Function  TreatAsAtomicUnit=on
  MATLAB Function5 : MATLAB Function  TreatAsAtomicUnit=on
  Math Function : Math  Operator=transpose  SaturateOnIntegerOverflow=on
  Mux : Mux  Inputs=3
  Product : Product  Multiplication=Matrix(*)
  pitch_rate_d : Scope  NumInputPorts=2
  roll_rate_d : Scope  NumInputPorts=2
  yaw_rate_d : Scope  NumInputPorts=2
  Rd rated : Outport
  Rd rated1 : Outport  Port=2
  Rd rated2 : Outport  Port=3
  wires:
  Discrete Derivative3/1 -> yaw_rate_d/2, Mux/3
  MATLAB Function3/2(theta) -> Display11/1
  Discrete Derivative1/1 -> roll_rate_d/2, Mux/1
  Discrete Derivative2/1 -> pitch_rate_d/2, Mux/2
  Product/1 -> MATLAB Function5/1(A), Display6/1
  Discrete Derivative/1 -> Product/2, Display5/1
  MATLAB Function1/1(R) -> Rd rated/1, MATLAB Function3/1(R), Display9/1, Math Function/1, Discrete Derivative/1  "Rd"
  MATLAB Function3/1(phi) -> Display10/1
  MATLAB Function3/3(psi) -> Display12/1
  Math Function/1 -> Product/1, Display4/1
  MATLAB Function5/1(t) -> Demux3/1, Display8/1  "rated"
  Demux3/3 -> yaw_rate_d/1  "yaw_rate_d"
  Demux3/1 -> roll_rate_d/1  "roll_rate_d"
  Demux3/2 -> pitch_rate_d/1  "pitch_rate_d"
  Roll_d/1 -> Discrete Derivative1/1, MATLAB Function1/1(phi)
  ? -> MATLAB Function5/2(force)
  Yaw_d/1 -> Discrete Derivative3/1, MATLAB Function1/3(psi)
  PItch_d/1 -> Discrete Derivative2/1, MATLAB Function1/2(theta)
  Discrete Derivative4/1 -> Rd rated2/1  "ratedd"
  Mux/1 -> Rd rated1/1, Discrete Derivative4/1

== matlab function multi_model/control_system1/Subsystem/MATLAB Function3 ==
  data: angular input; R output
function R = RPY_2_ZXY(angular)
%written by Daniel Mellinger
phi=angular(1);theta=angular(2);psi=angular(3);
% BRW = [ cos(psi)*cos(theta) - sin(phi)*sin(psi)*sin(theta), 
%     cos(theta)*sin(psi) + cos(psi)*sin(phi)*sin(theta), -cos(phi)*sin(theta)]
% 
% [                                 -cos(phi)*sin(psi),
%     cos(phi)*cos(psi),             sin(phi)]
% 
% [ cos(psi)*sin(theta) + cos(theta)*sin(phi)*sin(psi), 
%     sin(psi)*sin(theta) - cos(psi)*cos(theta)*sin(phi),
%     cos(phi)*cos(theta)]

R = [ cos(psi)*cos(theta) - sin(phi)*sin(psi)*sin(theta),... 
    cos(theta)*sin(psi) + cos(psi)*sin(phi)*sin(theta), -cos(phi)*sin(theta);...
    -cos(phi)*sin(psi),...
    cos(phi)*cos(psi),             sin(phi);...
    cos(psi)*sin(theta) + cos(theta)*sin(phi)*sin(psi),...
    sin(psi)*sin(theta) - cos(psi)*cos(theta)*sin(phi),...
    cos(phi)*cos(theta)];
    
    R = R';

== matlab function multi_model/control_system1/Subsystem3/R_c-and-Omega/MATLAB Function5 ==
  data: A input; t output; force input
function t = vee_map(A, force)
    if(nargin == 1)
        force = false ;
    end
    if(~force)
        if(double(sum(abs(diag(A)))) > 1e-2)
            disp('Error in vee_map() - Nonzero diagonal') ;
%             keyboard ;
        end
    end
    %A = [0 -t(3) t(2) ; t(3) 0 -t(1) ; -t(2) t(1) 0] ;
    t = [A(3,2) ;
         A(1,3) ;
         A(2,1)] ;
end

== matlab function multi_model/control_system1/Subsystem3/MATLAB Function1 ==
  data: position_c input; A output; velocity_c input
function A  = position_attitude(position_c,velocity_c)
%输入包括两部分，当前状态和期望状态
%其中，
%当前状态有18个：当前位置position_c,当前速度velocity_c,当前角度attitude_c，当前角速度angular_velocity_c
%期望状态有：position_d = [0;02;02];velocity_d = [0;0;0];accleration_d = [0;0;0];

%%%%%%%%%%%%%%%%%%%%%%%%%%%%%%%%  Control  %%%%%%%%%%%%%%%%%
%%四旋翼参数
mQ = 0.26;g = 9.81 ;e1 = [1;0;0];e2 = [0;1;0];e3 = [0;0;1];
%  J = diag([0.00080, 0.00065, 0.0014]);
%%期望状态量
position_d = [0;0;-5];velocity_d = [0;0;0];accleration_d = [0;0;0];
%%%%%  位置控制
 e_p = position_c - position_d;
 e_v = velocity_c - velocity_d;

%  epsilon_bar = 4.5;
epsilon_bar = 4.5;
 kp_xy = 0.3/epsilon_bar^2 ;
 kd_xy = 0.6/epsilon_bar ;
 k1 = diag([kp_xy kp_xy 2]) ;
 k2 = diag([kd_xy kd_xy 1.5]) ;
 A =-(-k1*e_p - k2*e_v - mQ*g*e3+mQ*accleration_d);

== matlab function multi_model/control_system1/Subsystem/MATLAB Function4 ==
  data: angular input; R output
function R = RPY_2_ZXY(angular)
%written by Daniel Mellinger
phi=angular(1);theta=angular(2);psi=angular(3);
% BRW = [ cos(psi)*cos(theta) - sin(phi)*sin(psi)*sin(theta), 
%     cos(theta)*sin(psi) + cos(psi)*sin(phi)*sin(theta), -cos(phi)*sin(theta)]
% 
% [                                 -cos(phi)*sin(psi),
%     cos(phi)*cos(psi),             sin(phi)]
% 
% [ cos(psi)*sin(theta) + cos(theta)*sin(phi)*sin(psi), 
%     sin(psi)*sin(theta) - cos(psi)*cos(theta)*sin(phi),
%     cos(phi)*cos(theta)]

R = [ cos(psi)*cos(theta) - sin(phi)*sin(psi)*sin(theta),... 
    cos(theta)*sin(psi) + cos(psi)*sin(phi)*sin(theta), -cos(phi)*sin(theta);...
    -cos(phi)*sin(psi),...
    cos(phi)*cos(psi),             sin(phi);...
    cos(psi)*sin(theta) + cos(theta)*sin(phi)*sin(psi),...
    sin(psi)*sin(theta) - cos(psi)*cos(theta)*sin(phi),...
    cos(phi)*cos(theta)];
    
    R = R';

== matlab function multi_model/dynamic_model/LiPo Battery ==
  data: load input; voltage output; cell_voltage output
function [voltage, cell_voltage]= LiPo(load)

%================================Constants=================================

delta_t = 0.004;
max_current = 5.500;                % maximum current per motor             (A)
aux_current = 0.100;                % current of auxillary components       (A)        
capacity = 1.000;                   % LiPo current capacity                 (Ah)                                 
cells = 2;                          % LiPo cell count

%==========================================================================

persistent discharge;

if isempty(discharge)
    discharge = 0;
end

current = sum(max_current .* load.^2) + aux_current;
discharge = current * (delta_t / 3600) + discharge;

discharge_capacity = discharge / capacity;

if (0 < discharge_capacity) && (discharge_capacity <=0.20)
    cell_voltage = -14.029*discharge_capacity^3 + 16.975*discharge_capacity^2 - 5.3339*discharge_capacity + 4.2;
elseif (0.20 < discharge_capacity) && (discharge_capacity < 0.70)
    cell_voltage = -0.2*discharge_capacity + 3.74;
else
    cell_voltage = -48*discharge_capacity^3 + 89.6*discharge_capacity^2 - 55.08*discharge_capacity + 14.716;
end

if cell_voltage < (5 / cells)
    cell_voltage = 0;
end
cell_voltage = 4.2;
supply_voltage = cells * cell_voltage;
voltage = supply_voltage .* load;

%==========================================================================

== matlab function multi_model/dynamic_model/MATLAB Function ==
  data: roll input; pitch input; altitude input; sonar_alt output
function sonar_alt = ultrasonic(roll, pitch, altitude)
if altitude > 0
    sonar_alt = sqrt(altitude^2 + (sqrt((altitude*tan(roll))^2 + (altitude*tan(pitch))^2))^2);
else
    sonar_alt = 0;
end

== matlab function multi_model/dynamic_model/multicopter ==
  data: omega input; DCM input; velocity input; density input; rotors input; forces output; moments output
function [forces, moments] = multicopter(omega, DCM, velocity, density, rotors)

%================================Constants=================================

coefficient_drag = 15;              % coefficient of drag
rotor_inertia = 0.0000025;          % rotor inertia                         (kg m^2)
prop_diameter = 0.1397;             % diameter of the propellor             (meters)                                 
% aircraft_mass = 0.26;               % aircraft mass                         (kg) 
aircraft_mass = 0.26; 
aircraft_diameter = 0.25;           % motor to motor distance               (meters)                                      

%==============================Actuator Mixer==============================

% [x(roll), y(pitch), z(yaw)]


MIX = [  1   1  -1   ;      % QUAD [X]
        -1   1   1   ;
        -1  -1  -1   ;
         1  -1   1   ;
         0   0   0   ;
         0   0   0   ;
         0   0   0   ;
         0   0   0   ];

% MIX = [  0   1  -1   ;      % QUAD [+]
%         -1   0   1   ;
%          0  -1  -1   ;
%          1   0   1   ;
%          0   0   0   ;
%          0   0   0   ;
%          0   0   0   ;
%          0   0   0   ];

% MIX = [  1   1  -1   ;      % HEX [X]
%         -1   1   1   ;
%         -1   0  -1   ;
%         -1  -1   1   ;
%          1  -1  -1   ;
%          1   0   1   ;
%          0   0   0   ;
%          0   0   0   ];

%==================================Forces================================== 

a = [   aircraft_diameter^2 / 10                        ;...                % body cross sectional area (X)
        aircraft_diameter^2 / 10                        ;...                % body cross sectional area (Y)
        sum(abs(MIX(:, 3))) * pi/4 * prop_diameter^2    ];                  % body cross sectional area (Z)
    
gravity = aircraft_mass .* (DCM * [0; 0; 9.81]);                            % gravitational force
% drag = -velocity .* coefficient_drag .* density .* a;                       % drag force
drag = [0;0;0];
%--------------------------------Thrust Model------------------------------
thrust = abs(MIX(:, 3)) .* (1*1E-3) .* rotors;                              % rotor thrust <==     
%--------------------------------------------------------------------------

forces = gravity + drag;
forces(3) = forces(3) - sum(thrust);

%==================================Moments=================================

mx = thrust .* MIX(:,1) .* (aircraft_diameter / 2)*sind(45);                % x moment
my = thrust .* MIX(:,2) .* (aircraft_diameter / 2)*sind(45);                % y moment

momentum_x = sum(abs(MIX(:, 3)) .* rotor_inertia .* rotors) * omega(1);     % x rotor momentum
momentum_y = sum(abs(MIX(:, 3)) .* rotor_inertia .* rotors) * omega(2);     % y rotor momentum
momentum_z = sum(MIX(:, 3) .* rotor_inertia .* rotors) * omega(3);          % z rotor momentum

%--------------------------------Torque Model------------------------------
mz = MIX(:,3) .* (1.7E-5) .* rotors;                                        % rotor torque <==
%--------------------------------------------------------------------------

% moments = [sum(mx); sum(my); sum(mz)] - [momentum_x; momentum_y;
% momentum_z];%%momented by yike
moments = [sum(mx); sum(my); sum(mz)];%%added by yike

%==========================================================================

== matlab function multi_model/control_system1/Subsystem/MATLAB Function5 ==
  data: RdR_RRd input; err_R output
function err_R = vee(RdR_RRd)
%     if(nargin == 1)
%         force = false ;
%     end
%     if(~force)
%         if(double(sum(abs(diag(A)))) > 1e-2)
%             disp('Error in vee_map() - Nonzero diagonal') ;
% %             keyboard ;
%         end
%     end
    %A = [0 -t(3) t(2) ; t(3) 0 -t(1) ; -t(2) t(1) 0] ;
    err_R = [RdR_RRd(3,2) ;
         RdR_RRd(1,3) ;
         RdR_RRd(2,1)] ;
end

== matlab function multi_model/control_system1/Subsystem/MATLAB Function7 ==
  data: a input; RR output; b input
function RR = a_b(a,b)
RR = a'*b ;

== matlab function multi_model/control_system1/Subsystem/MATLAB Function8 ==
  data: a input; RR output; b input
function RR = a_b(a,b)
RR = a'*b ;

== matlab function multi_model/control_system1/Subsystem/MATLAB Function1 ==
  data: phi input; R output; theta input; psi input
function R = RPYtoRot_ZXY(phi,theta,psi)
%written by Daniel Mellinger

% BRW = [ cos(psi)*cos(theta) - sin(phi)*sin(psi)*sin(theta), 
%     cos(theta)*sin(psi) + cos(psi)*sin(phi)*sin(theta), -cos(phi)*sin(theta)]
% 
% [                                 -cos(phi)*sin(psi),
%     cos(phi)*cos(psi),             sin(phi)]
% 
% [ cos(psi)*sin(theta) + cos(theta)*sin(phi)*sin(psi), 
%     sin(psi)*sin(theta) - cos(psi)*cos(theta)*sin(phi),
%     cos(phi)*cos(theta)]

R = [ cos(psi)*cos(theta) - sin(phi)*sin(psi)*sin(theta),... 
    cos(theta)*sin(psi) + cos(psi)*sin(phi)*sin(theta), -cos(phi)*sin(theta);...
    -cos(phi)*sin(psi),...
    cos(phi)*cos(psi),             sin(phi);...
    cos(psi)*sin(theta) + cos(theta)*sin(phi)*sin(psi),...
    sin(psi)*sin(theta) - cos(psi)*cos(theta)*sin(phi),...
    cos(phi)*cos(theta)];
    
    R = R';

== matlab function multi_model/control_system1/Subsystem3/MATLAB Function2 ==
  data: A input; M_roll output; R input; angular_velocity_c input; M_pitch output; M_yaw output; u1 output; rolld output; pitchd output; yawd output; Rd output; kR output; kOm output; Rd input; err_R output; err_Om output; rated input; ratedd input; psi_attract output; kR_test input; kOm_test input
function [M_roll, M_pitch,M_yaw,u1,rolld,pitchd,yawd,Rd,kR,kOm,err_R,err_Om,psi_attract] = attitude(A,R,angular_velocity_c,Rd,rated,ratedd,kR_test,kOm_test)

 J = diag([0.00080, 0.00065, 0.0014]);
 J_ni=inv(J);
 e1 = [1;0;0];e2 = [0;1;0];e3 = [0;0;1];

Omega=angular_velocity_c;

Omegad = rated;
dOmegad = ratedd;

 b3c = A/norm(A);
 b3 = R(:,3);
 f = vec_dot(A,b3);
 u1=f;
    
%%%%%  姿态控制
 b1d = e1;
 b1c = -vec_cross(b3c,vec_cross(b3c,b1d));
 b1c = b1c/norm(vec_cross(b3c,b1d));
 Rc = [b1c vec_cross(b3c,b1c) b3c];
 Rd=Rc;

[rolld,pitchd,yawd]=RotToRPY_ZXY(Rd);
 if(norm(Rd'*Rd-eye(3)) > 1e-2)
        disp('Error in R') ;
 end

%  kR = 0.4 ; kOm = 0.4 ;
%   kR = 3	 ; kOm =2 ;
%   kR = 0.09	 ; kOm =1 ;
kR = 0.5	 ; kOm =0.1;
kR=kR_test;kOm=kOm_test;
% epsilon = 0.1 ; %.5 ; %0.01 ;

psi_attract = 1/2*trace(eye(3,3)-Rd'*R);
err_R = 1/2 * vee_map(Rd'*R - R'*Rd) ;
err_Om = Omega - R'*Rd*Omegad ;
 

M = -kR.*err_R - kOm.*err_Om+ vec_cross(Omega, J*Omega)- J*(hat_map(Omega)*R'*Rd*Omegad - R'*Rd*dOmegad) ;
%  M = -kR.*err_R - kOm.*err_Om ;
M_roll=M(1);M_pitch=M(2);M_yaw=M(3);

== matlab function multi_model/control_system1/Subsystem3/MATLAB Function4 ==
  data: R input; phi output; theta output; psi output
function [phi,theta,psi] = RotToRPY_ZXY(R)
%written by Daniel Mellinger

% 
% R = [ cos(psi)*cos(theta) - sin(phi)*sin(psi)*sin(theta), 
%     cos(theta)*sin(psi) + cos(psi)*sin(phi)*sin(theta), -cos(phi)*sin(theta)]
% 
% [                                 -cos(phi)*sin(psi),
%     cos(phi)*cos(psi),             sin(phi)]
% 
% [ cos(psi)*sin(theta) + cos(theta)*sin(phi)*sin(psi), 
%     sin(psi)*sin(theta) - cos(psi)*cos(theta)*sin(phi),  cos(phi)*cos(theta)]
R = R';
phi = asin(R(2,3));
psi = atan2(-R(2,1)/cos(phi),R(2,2)/cos(phi));
theta = atan2(-R(1,3)/cos(phi),R(3,3)/cos(phi));
